simulink model "ACDS443_Prop"  (R2018b)
settings: Solver=VariableStepAuto  StartTime=0.0  StopTime=6000  RelTol=1e-3
model workspace (MAT data in the model file):
  NormalVec = Simulink.NumericType
  NormalVec.DataTypeMode = 'Double'
  NormalVec.SignednessBool = 1
  NormalVec.WordLength = 64
  NormalVec.FixedExponent = 0
  NormalVec.SlopeAdjustmentFactor = 1
  NormalVec.Bias = 0
  NormalVec.DataTypeOverride = 'Inherit'
  NormalVec.IsAlias = 0
  NormalVec.DataScope = 'Auto'
libraries: shared6dof x1
settings Model: Creator=atnguye2  LastModifiedBy=atnguye2

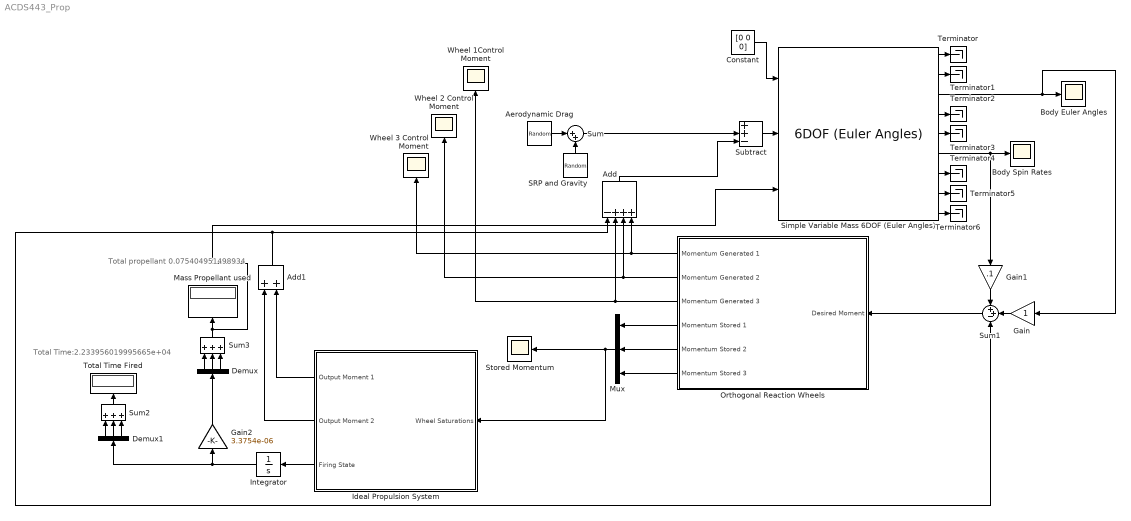
== system ACDS443_Prop ==
  note: Total Time:2.233956019995665e+04
  note: Total propellant 0.075404951498934
  Add : Sum  Inputs=-+++
  Add1 : Sum
  Aerodynamic Drag : RandomNumber  Mean=[0 0 0]  Variance=[1 1 1]*6.34e-11  Seed=1:3  SampleTime=0.1  VectorParams1D=off
  Body Euler Angles : Scope
  Body Spin Rates : Scope
  Constant : Constant  Value=[0 0 0]
  Demux : Demux  Outputs=3
  Demux1 : Demux  Outputs=3
  Gain : Gain
  Gain1 : Gain  Gain=.1
  Gain2 : Gain  Gain=3.3754e-06
  Ideal Propulsion System : Subsystem
      mask Display: image('\\ad.uillinois.edu\engr-ews\atnguye2\Downloads\large.png');
  Integrator : Integrator
  Mass Propellant used : Display
  Mux : Mux  Inputs=3
  Orthogonal Reaction Wheels : Subsystem
      mask Display: image('\\ad.uillinois.edu\engr-ews\atnguye2\Documents\My Pictures\Capture.PNG');
  "SRP and Gravity " : RandomNumber  Mean=[0 0 0]  Variance=[1 1 1]*1.3*10^-8  Seed=1:3  SampleTime=0.1  VectorParams1D=off
  Simple Variable Mass 6DOF (Euler Angles) : shared6dof/6DOF (Euler Angles)  units=Metric (MKS)  mtype=Simple Variable  rep=Euler Angles  xme_0=[0 0 0]  Vm_0=[0 0 0]  eul_0=[0 0 0]  pm_0=[0.174533 0.174533 0.174533]  mass_0=1.0  mass_e=0.5  mass_f=2.0  inertia=eye(3)  inertia_e=zeros(3)  inertia_f="diag([0.0541, 0.1054,  0.0914])"  k_quat=1.0  vre_flag=off  abi_flag=off  aMode=0  xme_statename={'Xe', 'Ye', 'Ze'}  Vm_statename={'U', 'v', 'w'}  eul_statename={'phi', 'theta', 'psi'}  quat_statename=''  pm_statename={'p', 'q', 'r'}  mass_statename='mass'
      settings: SourceProductBaseCode=AE
  Stored Momentum : Scope
  Subtract : Sum  Inputs=++-
  Sum : Sum  Inputs=|++
  Sum1 : Sum  Inputs=++-
  Sum2 : Sum  Inputs=3
  Sum3 : Sum  Inputs=3
  Terminator{,1..6} (7 alike) : Terminator
  Total Time Fired : Display
  Wheel 1Control Moment : Scope
  "Wheel 2 Control Moment " : Scope
  Wheel 3 Control Moment : Scope
  wires:
  Sum3/1 -> Simple Variable Mass 6DOF (Euler Angles)/3, Mass Propellant used/1
  Aerodynamic Drag/1 -> Sum/1
  "SRP and Gravity "/1 -> Sum/2
  Constant/1 -> Simple Variable Mass 6DOF (Euler Angles)/1
  Subtract/1 -> Simple Variable Mass 6DOF (Euler Angles)/2
  Add/1 -> Subtract/3
  Mux/1 -> Ideal Propulsion System/1(Wheel Saturations), Stored Momentum/1
  Sum1/1 -> Orthogonal Reaction Wheels/1(Desired Moment)
  Orthogonal Reaction Wheels/4(Momentum Stored 1) -> Mux/1
  Orthogonal Reaction Wheels/5(Momentum Stored 2) -> Mux/2
  Orthogonal Reaction Wheels/6("Momentum Stored 3 ") -> Mux/3
  Orthogonal Reaction Wheels/1(Momentum Generated 1) -> Wheel 3 Control Moment/1, Add/4
  Add1/1 -> Add/1, Sum1/3
  Demux/1 -> Sum3/1
  Demux/2 -> Sum3/2
  Demux/3 -> Sum3/3
  Gain2/1 -> Demux/1
  Ideal Propulsion System/2(Output Moment 2) -> Add1/1
  Ideal Propulsion System/1(Output Moment 1) -> Add1/2
  Demux1/2 -> Sum2/2
  Demux1/1 -> Sum2/1
  Ideal Propulsion System/3(Firing State) -> Integrator/1
  Demux1/3 -> Sum2/3
  Sum2/1 -> Total Time Fired/1
  Orthogonal Reaction Wheels/2(Momentum Generated 2) -> "Wheel 2 Control Moment "/1, Add/3
  Orthogonal Reaction Wheels/3("Momentum Generated 3 ") -> Wheel 1Control Moment/1, Add/2
  Simple Variable Mass 6DOF (Euler Angles)/3 -> Gain/1, Body Euler Angles/1
  Integrator/1 -> Demux1/1, Gain2/1
  Sum/1 -> Subtract/2
  Simple Variable Mass 6DOF (Euler Angles)/6 -> Body Spin Rates/1, Gain1/1
  Gain/1 -> Sum1/2
  Gain1/1 -> Sum1/1
  Simple Variable Mass 6DOF (Euler Angles)/1 -> Terminator/1
  Simple Variable Mass 6DOF (Euler Angles)/2 -> Terminator1/1
  Simple Variable Mass 6DOF (Euler Angles)/4 -> Terminator2/1
  Simple Variable Mass 6DOF (Euler Angles)/5 -> Terminator3/1
  Simple Variable Mass 6DOF (Euler Angles)/7 -> Terminator4/1
  Simple Variable Mass 6DOF (Euler Angles)/8 -> Terminator5/1
  Simple Variable Mass 6DOF (Euler Angles)/9 -> Terminator6/1

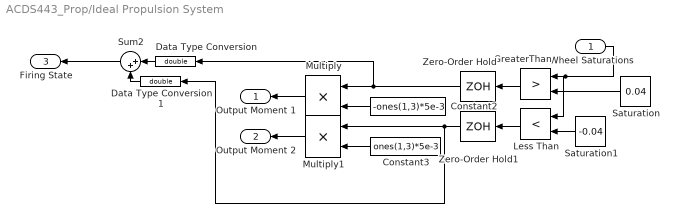
== system ACDS443_Prop/Ideal Propulsion System ==
  Wheel Saturations : Inport
  Constant2 : Constant  Value=-ones(1,3)*5e-3
  Constant3 : Constant  Value=ones(1,3)*5e-3
  Data Type Conversion : DataTypeConversion  OutDataTypeStr=double
  Data Type Conversion1 : DataTypeConversion  OutDataTypeStr=double
  GreaterThan : RelationalOperator  Operator=>  OutDataTypeStr=boolean  RndMeth=Simplest
  Less Than : RelationalOperator  Operator=<  OutDataTypeStr=boolean  RndMeth=Simplest
  Multiply : Product
  Multiply1 : Product
  Saturation : Constant  Value=0.04
  Saturation1 : Constant  Value=-0.04
  Sum2 : Sum  Inputs=|++
  Zero-Order Hold : ZeroOrderHold  SampleTime=8
  Zero-Order Hold1 : ZeroOrderHold  SampleTime=8
  Output Moment 1 : Outport
  Output Moment 2 : Outport  Port=2
  Firing State : Outport  Port=3
  wires:
  Saturation1/1 -> Less Than/2
  Zero-Order Hold1/1 -> Multiply1/1, Data Type Conversion1/1
  Data Type Conversion1/1 -> Sum2/2
  Constant2/1 -> Multiply/2
  Data Type Conversion/1 -> Sum2/1
  Saturation/1 -> GreaterThan/2
  Less Than/1 -> Zero-Order Hold1/1
  Constant3/1 -> Multiply1/2
  Multiply1/1 -> Output Moment 2/1
  Zero-Order Hold/1 -> Data Type Conversion/1, Multiply/1
  GreaterThan/1 -> Zero-Order Hold/1
  Wheel Saturations/1 -> Less Than/1, GreaterThan/1
  Multiply/1 -> Output Moment 1/1
  Sum2/1 -> Firing State/1

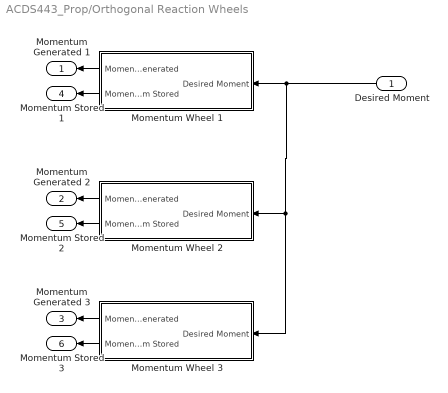
== system ACDS443_Prop/Orthogonal Reaction Wheels ==
  Desired Moment : Inport
  Momentum Wheel 1 : Subsystem  mask{NormalVector=[1 0 0]}
      mask prompts: NormalVector "What is the wheel's orientation"
  Momentum Wheel 2 : Subsystem  mask{NormalVector=[0 1 0]}
      mask prompts: NormalVector "What is the wheel's orientation"
  Momentum Wheel 3 : Subsystem  mask{NormalVector=[0 0 1]}
      mask prompts: NormalVector "What is the wheel's orientation"
  Momentum Generated 1 : Outport
  Momentum Generated 2 : Outport  Port=2
  "Momentum Generated 3 " : Outport  Port=3
  Momentum Stored 1 : Outport  Port=4
  Momentum Stored 2 : Outport  Port=5
  "Momentum Stored 3 " : Outport  Port=6
  wires:
  Momentum Wheel 2/2(Momentum Stored) -> Momentum Stored 2/1
  Momentum Wheel 2/1("Momentum Generated ") -> Momentum Generated 2/1
  Desired Moment/1 -> Momentum Wheel 3/1(Desired Moment), Momentum Wheel 2/1(Desired Moment), Momentum Wheel 1/1(Desired Moment)
  Momentum Wheel 3/1("Momentum Generated ") -> "Momentum Generated 3 "/1
  Momentum Wheel 3/2(Momentum Stored) -> "Momentum Stored 3 "/1
  Momentum Wheel 1/1("Momentum Generated ") -> Momentum Generated 1/1
  Momentum Wheel 1/2(Momentum Stored) -> Momentum Stored 1/1

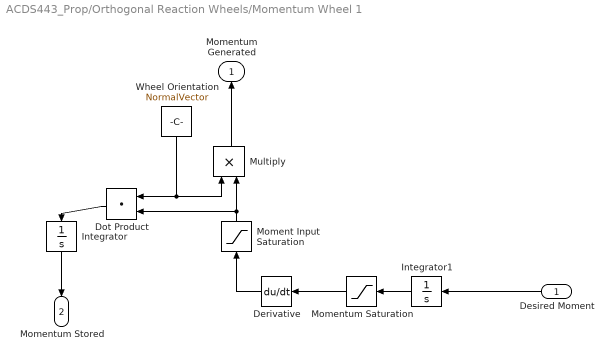
== system ACDS443_Prop/Orthogonal Reaction Wheels/Momentum Wheel 1 ==
  Desired Moment : Inport
  Derivative : Derivative
  Dot Product : DotProduct  InputSameDT=on  OutDataTypeStr=Inherit: Inherit via internal rule
  Integrator : Integrator  InitialCondition=.037
  Integrator1 : Integrator
  Moment Input Saturation : Saturate  UpperLimit=20e-3  LowerLimit=-20e-3  LinearizeAsGain=off
  Momentum Saturation : Saturate  UpperLimit=.05  LowerLimit=-.05
  Multiply : Product
  Wheel Orientation : Constant  Value=NormalVector
  "Momentum Generated " : Outport
  Momentum Stored : Outport  Port=2
  wires:
  Integrator1/1 -> Momentum Saturation/1
  Derivative/1 -> Moment Input Saturation/1
  Momentum Saturation/1 -> Derivative/1
  Desired Moment/1 -> Integrator1/1
  Moment Input Saturation/1 -> Dot Product/2, Multiply/2
  Multiply/1 -> "Momentum Generated "/1
  Wheel Orientation/1 -> Dot Product/1, Multiply/1
  Integrator/1 -> Momentum Stored/1
  Dot Product/1 -> Integrator/1

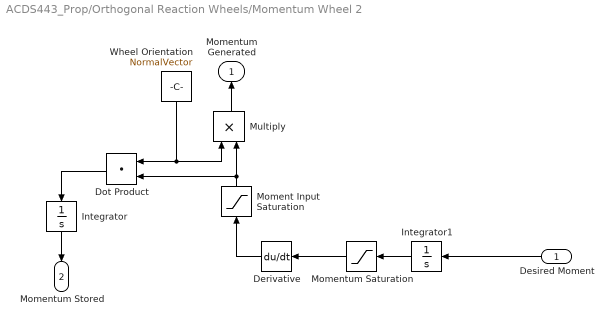
== system ACDS443_Prop/Orthogonal Reaction Wheels/Momentum Wheel 2 ==
  Desired Moment : Inport
  Derivative : Derivative
  Dot Product : DotProduct  InputSameDT=on  OutDataTypeStr=Inherit: Inherit via internal rule
  Integrator : Integrator
  Integrator1 : Integrator
  Moment Input Saturation : Saturate  UpperLimit=20e-3  LowerLimit=-20e-3  LinearizeAsGain=off
  Momentum Saturation : Saturate  UpperLimit=.05  LowerLimit=-.05
  Multiply : Product
  Wheel Orientation : Constant  Value=NormalVector
  "Momentum Generated " : Outport
  Momentum Stored : Outport  Port=2
  wires:
  Integrator1/1 -> Momentum Saturation/1
  Derivative/1 -> Moment Input Saturation/1
  Momentum Saturation/1 -> Derivative/1
  Desired Moment/1 -> Integrator1/1
  Moment Input Saturation/1 -> Dot Product/2, Multiply/2
  Multiply/1 -> "Momentum Generated "/1
  Wheel Orientation/1 -> Dot Product/1, Multiply/1
  Integrator/1 -> Momentum Stored/1
  Dot Product/1 -> Integrator/1

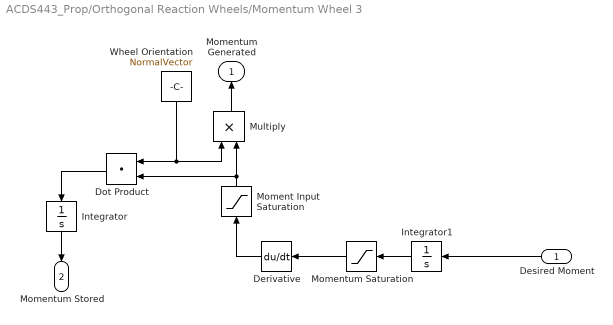
== system ACDS443_Prop/Orthogonal Reaction Wheels/Momentum Wheel 3 ==
  Desired Moment : Inport
  Derivative : Derivative
  Dot Product : DotProduct  InputSameDT=on  OutDataTypeStr=Inherit: Inherit via internal rule
  Integrator : Integrator
  Integrator1 : Integrator
  Moment Input Saturation : Saturate  UpperLimit=20e-3  LowerLimit=-20e-3  LinearizeAsGain=off
  Momentum Saturation : Saturate  UpperLimit=.05  LowerLimit=-.05
  Multiply : Product
  Wheel Orientation : Constant  Value=NormalVector
  "Momentum Generated " : Outport
  Momentum Stored : Outport  Port=2
  wires:
  Integrator1/1 -> Momentum Saturation/1
  Derivative/1 -> Moment Input Saturation/1
  Momentum Saturation/1 -> Derivative/1
  Desired Moment/1 -> Integrator1/1
  Moment Input Saturation/1 -> Dot Product/2, Multiply/2
  Multiply/1 -> "Momentum Generated "/1
  Wheel Orientation/1 -> Dot Product/1, Multiply/1
  Integrator/1 -> Momentum Stored/1
  Dot Product/1 -> Integrator/1
